simulink model "example212s"  (R2023b)
settings: Solver=ode4  StartTime=0.0  StopTime=10  FixedStep=0.1  RelTol=1e-3
libraries: simulink x1
settings Model: Creator=GPL  LastModifiedBy=17547
settings SolverCC: AlgebraicLoopSolver=TrustRegion
settings DataIOCC: ReturnWorkspaceOutputs=off
settings DebuggingCC: UnconnectedInputMsg=warning  UnconnectedOutputMsg=warning  UnconnectedLineMsg=warning  ArithmeticOperatorsInVariantConditions=warning
settings ModelReferenceCC: EnableRefExpFcnMdlSchedulingChecks=on
settings SFSimCC: SimUseLocalCustomCode=off  CustomCodeUndefinedFunction=UseInterfaceOnly
settings RTWCC: RTWUseLocalCustomCode=off

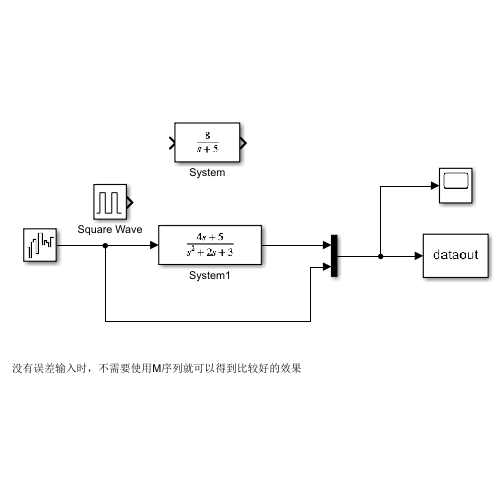
[thumbnail: Simulink's stored preview of the top-level diagram]
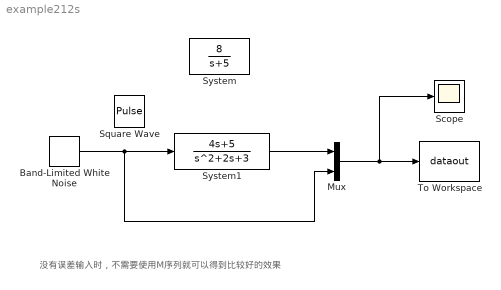
== system example212s ==
  note: 没有误差输入时，不需要使用M序列就可以得到比较好的效果
  Band-Limited White Noise : simulink/Sources/Band-Limited White Noise  Cov=[1]  Ts=0.1  seed=[23341]
  Mux : Mux  Inputs=2
  Scope : Scope
  Square Wave : DiscretePulseGenerator  PulseType=Time based  Period=5  PulseWidth=50
  System : TransferFcn  Numerator=[8]  Denominator=[1 5]  ContinuousStateAttributes='Plant'
  System1 : TransferFcn  Numerator=[4 5]  Denominator=[1 2 3 ]  ContinuousStateAttributes='Plant'
  To Workspace : ToWorkspace  VariableName=dataout  SaveFormat=Timeseries  SampleTime=-1
  wires:
  Band-Limited White Noise/1 -> System1/1, Mux/2
  System1/1 -> Mux/1
  Mux/1 -> Scope/1, To Workspace/1
